simulink subsystem "Sensors"  (R2024b)
settings: Solver=VariableStepAuto  StartTime=0.0  StopTime=10.0  RelTol=1e-3
undefined symbols (not defined in the file or in its folder): decyear, imu1_accel_bias, imu1_accel_noise, imu1_gyro_bias, imu1_gyro_noise, imu1_mag_noise, imu2_accel_bias, imu2_accel_noise, imu2_gyro_bias, imu2_gyro_noise, imu2_mag_noise, samplingrate
libraries: simulink x1
settings Model: Creator=joedo  LastModifiedBy=finnb

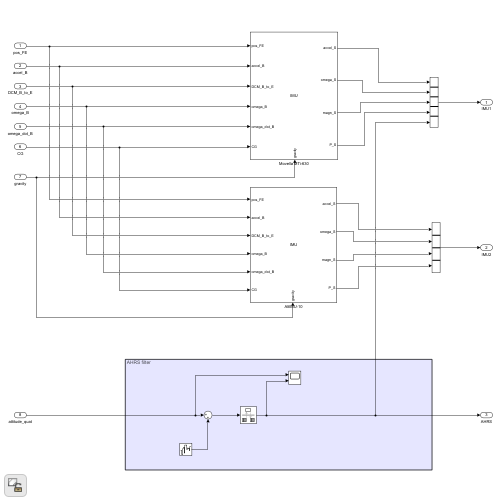
[thumbnail: Simulink's stored preview of the top-level diagram]
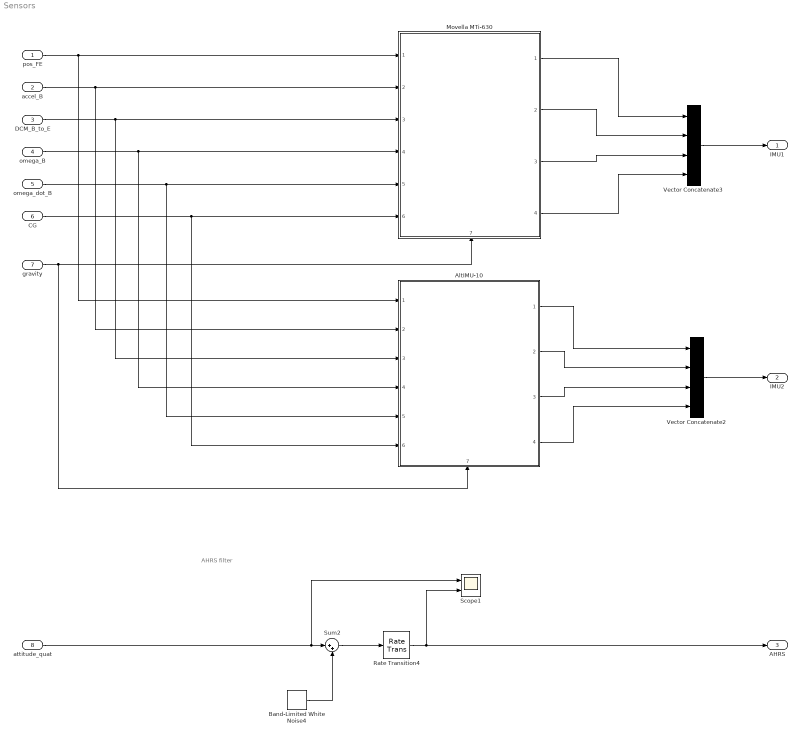
== system Sensors ==
  note: AHRS filter
  pos_FE : Inport
  accel_B : Inport  Port=2
  DCM_B_to_E : Inport  Port=3
  omega_B : Inport  Port=4
  omega_dot_B : Inport  Port=5
  CG : Inport  Port=6
  gravity : Inport  Port=7
  attitude_quat : Inport  Port=8
  AltIMU-10 : Subsystem  ReferencedSubsystem=IMU  noise_accel=imu2_accel_noise * [1 1 1]  bias_accel=imu2_accel_bias * (2*rand(3,1)-1)  scale_accel=eye(3)  lim_accel=imu2_accel_limit  noise_gyro=imu2_gyro_noise * [1 1 1]  bias_gyro=imu2_gyro_bias * (2*rand(3,1)-1)  scale_gyro=eye(3)  lim_gyro=imu2_gyro_limit  noise_mag=imu2_mag_noise * [1 1 1]  bias_mag=[0 0 0]  scale_mag=eye(3)  noise_pres=imu2_baro_noise  bias_pres=0  scale_pres=1  Ssi=sensor_2_S  Lsi=sensor_2_d  lon=80.5204  lat=43.4643  year=decyear(2025, 1,1)
      settings: PortSchema="{\"entries\":[{\"content\":{\"sides\":[{\"content\":{\"connectorIds\":[\"In1\",\"In2\",\"In3\",\"In4\",\"In5\",\"In6\"]},\"type\":\"ConnectorPlacement.EquallySpacedRectSide\",\"uuid\":\"7364b596-1fe2-4988-bcd1-f44de8b6ad1d\"},{\"content\":{\"connectorIds\":[\"Out1\",\"Out2\",\"Out3\",\"Out4\"],\"side\":\"RIGHT\"},\"type\":\"ConnectorPlacement.EquallySpacedRectSide\",\"uuid\":\"15b517ae-ede9-4e73-bdbe-ac90fe1cd4b3\"},{\"content\":{\"side\":\"TOP\"},\"type\":\"ConnectorPlacement.EquallySpacedRectSide\",\"uuid\":\"ed561e6a-ec50-4ee4-83d6-7eafc6eed540\"},{\"content\":{\"connectorIds\":[\"In7\"],\"side\":\"BOTTOM\"},\"type\":\"ConnectorPlacement.EquallySpacedRectSide\",\"uuid\":\"26459742-6ce2-4d6d-b6f5-2164d7913c5d\"}]},\"type\":\"ConnectorPlacement.EquallySpacedConnector\",\"uuid\":\"3eff0b54-08f9-4999-b05b-14bb156a91bd\"}],\"packageUris\":[\"http://schema.mathworks.com/mf0/Connector/R2020b\"],\"version\":\"1.0\"}"
  Band-Limited White Noise4 : simulink/Sources/Band-Limited White Noise  Cov=1e-4  Ts=samplingrate  seed=[2323451]
  Movella MTi-630 : Subsystem  ReferencedSubsystem=IMU  noise_accel=imu1_accel_noise * [1 1 1]  bias_accel=imu1_accel_bias * (2*rand(3,1)-1)  scale_accel=eye(3)  lim_accel=imu1_accel_limit  noise_gyro=imu1_gyro_noise * [1 1 1]  bias_gyro=imu1_gyro_bias * (2*rand(3,1)-1)  scale_gyro=eye(3)  lim_gyro=imu1_gyro_limit  noise_mag=imu1_mag_noise * [1 1 1]  bias_mag=[0 0 0]  scale_mag=eye(3)  noise_pres=imu1_baro_noise  bias_pres=0  scale_pres=1  Ssi=sensor_1_S  Lsi=sensor_1_d  lon=80.5204  lat=43.4643  year=decyear(2025, 1,1)
      settings: PortSchema="{\"entries\":[{\"content\":{\"sides\":[{\"content\":{\"connectorIds\":[\"In1\",\"In2\",\"In3\",\"In4\",\"In5\",\"In6\"]},\"type\":\"ConnectorPlacement.EquallySpacedRectSide\",\"uuid\":\"7364b596-1fe2-4988-bcd1-f44de8b6ad1d\"},{\"content\":{\"connectorIds\":[\"Out1\",\"Out2\",\"Out3\",\"Out4\"],\"side\":\"RIGHT\"},\"type\":\"ConnectorPlacement.EquallySpacedRectSide\",\"uuid\":\"15b517ae-ede9-4e73-bdbe-ac90fe1cd4b3\"},{\"content\":{\"side\":\"TOP\"},\"type\":\"ConnectorPlacement.EquallySpacedRectSide\",\"uuid\":\"ed561e6a-ec50-4ee4-83d6-7eafc6eed540\"},{\"content\":{\"connectorIds\":[\"In7\"],\"side\":\"BOTTOM\"},\"type\":\"ConnectorPlacement.EquallySpacedRectSide\",\"uuid\":\"26459742-6ce2-4d6d-b6f5-2164d7913c5d\"}]},\"type\":\"ConnectorPlacement.EquallySpacedConnector\",\"uuid\":\"3eff0b54-08f9-4999-b05b-14bb156a91bd\"}],\"packageUris\":[\"http://schema.mathworks.com/mf0/Connector/R2020b\"],\"version\":\"1.0\"}"
  Rate Transition4 : RateTransition  OutPortSampleTime=samplingrate
  Scope1 : Scope  NumInputPorts=2
  Sum2 : Sum  Inputs=|++
  Vector Concatenate2 : Concatenate  NumInputs=4
  Vector Concatenate3 : Concatenate  NumInputs=4
  IMU1 : Outport
  IMU2 : Outport  Port=2
  AHRS : Outport  Port=3
  wires:
  DCM_B_to_E/1 -> Movella MTi-630/3, AltIMU-10/3
  omega_B/1 -> AltIMU-10/4, Movella MTi-630/4
  AltIMU-10/3 -> Vector Concatenate2/3
  accel_B/1 -> Movella MTi-630/2, AltIMU-10/2
  pos_FE/1 -> Movella MTi-630/1, AltIMU-10/1
  AltIMU-10/4 -> Vector Concatenate2/4
  AltIMU-10/2 -> Vector Concatenate2/2
  AltIMU-10/1 -> Vector Concatenate2/1
  omega_dot_B/1 -> Movella MTi-630/5, AltIMU-10/5
  gravity/1 -> AltIMU-10/7, Movella MTi-630/7
  CG/1 -> AltIMU-10/6, Movella MTi-630/6
  Vector Concatenate2/1 -> IMU2/1
  Vector Concatenate3/1 -> IMU1/1
  Movella MTi-630/4 -> Vector Concatenate3/4
  Movella MTi-630/1 -> Vector Concatenate3/1
  Movella MTi-630/3 -> Vector Concatenate3/3
  Movella MTi-630/2 -> Vector Concatenate3/2
  Sum2/1 -> Rate Transition4/1
  Rate Transition4/1 -> AHRS/1, Scope1/2
  Band-Limited White Noise4/1 -> Sum2/2
  attitude_quat/1 -> Sum2/1, Scope1/1
